simulink model "vsi_square"  (R2020a)
settings: Solver=VariableStepAuto  StartTime=0.0  StopTime=1  RelTol=1e-3
undefined symbols (not defined in the file or in its folder): cfg
libraries: powerlib x22
settings Model: Creator=tomi_  LastModifiedBy=tomi_

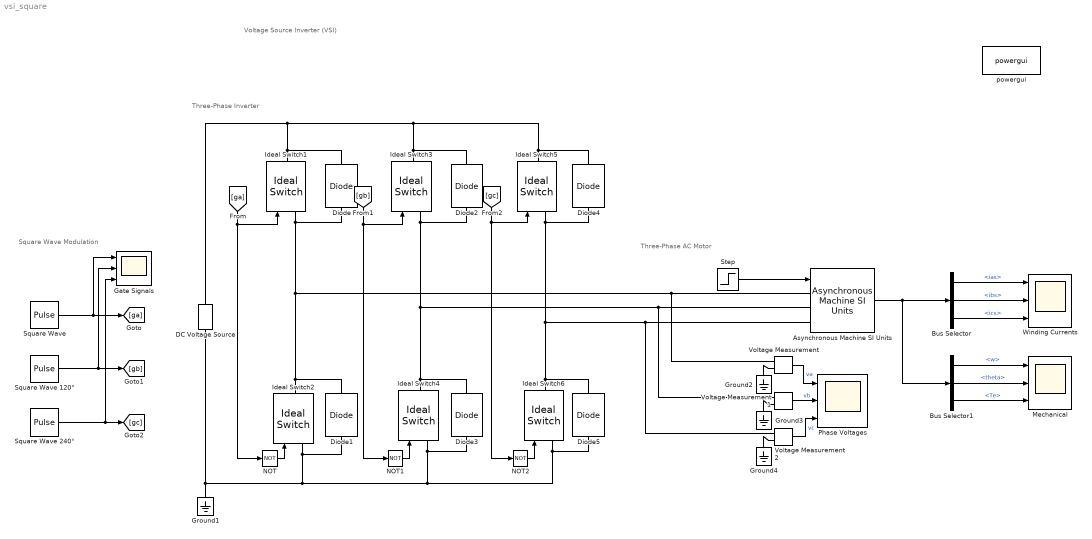
== system vsi_square ==
  note: Three-Phase AC Motor
  note: Three-Phase Inverter
  note: Square Wave Modulation
  note: Voltage Source Inverter (VSI)
  Asynchronous Machine SI Units : powerlib/Machines/Asynchronous Machine SI Units  RotorType=Squirrel-cage  PresetModel="01:  5 HP   460 V 60Hz 1750 RPM"  MechanicalLoad=Torque Tm  ShowDetailedParameters=on  ReferenceFrame=Synchronous  Units=SI  MeasurementBus=on  NominalParameters=[3730 460 60]  Stator=[1.115 0.005974]  Rotor=[1.083 0.005974]  Cage1=[0.4155 0.002066]  Cage2=[0.4168 0.0003495]  Lm=0.2037  Mechanical=[0.02 0.005752 2]  PolePairs=2  InitialConditions=[0 0 0 0 0 0 0 0]  SimulateSaturation=off  Saturation=[14.03593122, 27.81365428, 53.79336849, 72.68890987, 97.98006896, 148.6815601, 215.7428561, 302.9841135, 428.7778367 ; 230, 322, 414, 460, 506, 552, 598, 644, 690]  LoadFlowParameters=1492000  TsPowergui=0  TsBlock=-1  IterativeModel=Trapezoidal non iterative  IterativeDiscreteModel=Trapezoidal non iterative  Pmec=1.492e+006
  Bus Selector : BusSelector  OutputSignals=ias,ibs,ics
  Bus Selector1 : BusSelector  OutputSignals=w,theta,Te
  DC Voltage Source : powerlib/Electrical Sources/DC Voltage Source  Amplitude=cfg.vd  Measurements=None
  Diode{,1..5} (6 alike) : powerlib/Power Electronics/Diode  Ron=0.001  Lon=0  Vf=0  IC=0  UseSnubber=0  Rs=inf  Cs=250e-9  Measurements=off
  Gate Signals : Scope  NumInputPorts=3
  Ground{1..4} (4 alike) : powerlib/Elements/Ground  LConnTagsString=a
  Ideal Switch{1..6} (6 alike) : powerlib/Power Electronics/Ideal Switch  Ron=0.001  Lon=0  IC=0  Rs=inf  Cs=inf  Measurements=off
  Mechanical : Scope  NumInputPorts=3
  NOT : Logic  Operator=NOT  IconShape=distinctive  AllPortsSameDT=off  OutDataTypeStr=boolean
  NOT1 : Logic  Operator=NOT  IconShape=distinctive  AllPortsSameDT=off  OutDataTypeStr=boolean
  NOT2 : Logic  Operator=NOT  IconShape=distinctive  AllPortsSameDT=off  OutDataTypeStr=boolean
  Phase Voltages : Scope  NumInputPorts=3
  Square Wave : DiscretePulseGenerator  PulseType=Time based  Amplitude=cfg.ctrl.ampl  Period=1/cfg.ctrl.freq  PulseWidth=50
  Square Wave 120° : DiscretePulseGenerator  PulseType=Time based  Amplitude=cfg.ctrl.ampl  Period=1/cfg.ctrl.freq  PulseWidth=50  PhaseDelay=(120/360)/cfg.ctrl.freq
  Square Wave 240° : DiscretePulseGenerator  PulseType=Time based  Amplitude=cfg.ctrl.ampl  Period=1/cfg.ctrl.freq  PulseWidth=50  PhaseDelay=(240/360)/cfg.ctrl.freq
  Step : Step  Time=0.5  After=5  SampleTime=0
  Voltage Measurement : powerlib/Measurements/Voltage Measurement  PhasorSimulation=off  OutputType=Complex  PSBequivalent=0
  Voltage Measurement1 : powerlib/Measurements/Voltage Measurement  PhasorSimulation=off  OutputType=Complex  PSBequivalent=0
  Voltage Measurement2 : powerlib/Measurements/Voltage Measurement  PhasorSimulation=off  OutputType=Complex  PSBequivalent=0
  Winding Currents : Scope  NumInputPorts=3
  powergui : powerlib/powergui  Priority=1  SimulationMode=Continuous  SampleTime=50e-6  frequency=60  Iterations=50  frequencyindice=0  Pbase=100e6  ErrMax=1e-4  UnitsV=kV  UnitsW=MW  buscounter=0  FunctionMessages=off  echomessages=off  EnableUseOfTLC=off  CurrentSourceSwitches=off  DisableSnubberDevices=off  DisableRonSwitches=off  DisableVfSwitches=off  DisplayEquations=off  AutomaticDiscreteSolvers=off  SolverType=Tustin/Backward Euler (TBE)  Interpol=off  ExternalGateDelay=off  methode=off  Ts=100  x0status=blocks  SPID=on  SwTol=0  HookPort=off  NonlinearTolerance=1e-4  nMaxIteration=100  ContinueOnMaxIteration=off  RestoreLinks=warning  ResistiveCurrentMeasurement=off  Frange=[0:2:500]  Ylog=off  Xlog=on  ShowGrid=off  save=off  variable=ZData  structure=0  ZoomFFT=off  StartTime=0.0  cycles=1  DisplayStyle=1  fundamental=60  FreqAxis=off  MaxFrequency=1000  frequencyindicesteady=1  RmsSteady=1  display=off
  wires:
  Square Wave/1 -> Gate Signals/1, [ga]
  Square Wave 120°/1 -> Gate Signals/2, [gb]
  [ga] -> Ideal Switch1/1, NOT/1
  [gb] -> Ideal Switch3/1, NOT1/1
  [gc] -> Ideal Switch5/1, NOT2/1
  NOT/1 -> Ideal Switch2/1
  NOT1/1 -> Ideal Switch4/1
  NOT2/1 -> Ideal Switch6/1
  Voltage Measurement/1 -> Phase Voltages/1  "va"
  Voltage Measurement1/1 -> Phase Voltages/2  "vb"
  Voltage Measurement2/1 -> Phase Voltages/3  "vc"
  Bus Selector/1 -> Winding Currents/1  "<ias>"
  Bus Selector/3 -> Winding Currents/3  "<ics>"
  Step/1 -> Asynchronous Machine SI Units/1
  Bus Selector/2 -> Winding Currents/2  "<ibs>"
  Bus Selector1/3 -> Mechanical/3  "<Te>"
  Bus Selector1/2 -> Mechanical/2  "<theta>"
  Bus Selector1/1 -> Mechanical/1  "<w>"
  Asynchronous Machine SI Units/1 -> Bus Selector1/1, Bus Selector/1
  Square Wave 240°/1 -> Gate Signals/3, [gc]
  connections:
  Ideal Switch2/RConn1 -- Diode1/RConn1 -- Diode/LConn1 -- Ideal Switch1/LConn1 -- Asynchronous Machine SI Units/LConn1 -- Voltage Measurement/LConn1
  Ideal Switch4/RConn1 -- Diode3/RConn1 -- Diode2/LConn1 -- Ideal Switch3/LConn1 -- Asynchronous Machine SI Units/LConn2 -- Voltage Measurement1/LConn1
  Ideal Switch6/RConn1 -- Diode5/RConn1 -- Diode4/LConn1 -- Ideal Switch5/LConn1 -- Asynchronous Machine SI Units/LConn3 -- Voltage Measurement2/LConn1
  Ideal Switch2/LConn1 -- Diode1/LConn1 -- DC Voltage Source/LConn1 -- Ground1/LConn1 -- Diode3/LConn1 -- Ideal Switch4/LConn1 -- Diode5/LConn1 -- Ideal Switch6/LConn1
  Ideal Switch5/RConn1 -- Diode2/RConn1 -- Ideal Switch3/RConn1 -- Diode/RConn1 -- Ideal Switch1/RConn1 -- DC Voltage Source/RConn1 -- Diode4/RConn1
  Ground2/LConn1 -- Voltage Measurement/LConn2
  Ground3/LConn1 -- Voltage Measurement1/LConn2
  Ground4/LConn1 -- Voltage Measurement2/LConn2
